simulink model "duplointegrador_2020"  (R2020b)
settings: Solver=ode4  StartTime=0.0  StopTime=30  FixedStep=1e-3  RelTol=1e-3
values from neighbouring files (symbols this model uses):
  N = 4    [duplointegrador_plot_2020.m]
undefined symbols (not defined in the file or in its folder): C, DiscIntNeverNeededParam, Flqr, G, Gamma, h, n, Phi, Q, Q0, Q1, Q2, R, UM, Um, x10, x20, YM, Ym
libraries: simulink x6, eeLuenbergerObserver x1
settings Model: Creator=Trevor  LastModifiedBy=lucas
settings SolverCC: AutoInsertRateTranBlk=on
settings DataIOCC: LimitDataPoints=on  SaveFormat=Array  ReturnWorkspaceOutputs=off
settings OptimizationCC: LifeSpan=inf
settings DebuggingCC: SFUnexpectedBacktrackingDiag=warning  SFNoUnconditionalDefaultTransitionDiag=warning  SFExecutionAtInitializationDiag=none  ArithmeticOperatorsInVariantConditions=warning
settings HardwareCC: ProdBitPerPointer=32  ProdBitPerSizeT=32  ProdBitPerPtrDiffT=32  ProdLargestAtomicFloat=None  ProdIntDivRoundTo=Undefined  ProdEndianess=Unspecified  ProdWordSize=32  ProdHWDeviceType=32-bit Generic
settings ModelReferenceCC: PropagateSignalLabelsOutOfModel=off
settings SFSimCC: SimUseLocalCustomCode=off  CustomCodeUndefinedFunction=UseInterfaceOnly
settings RTWCC: RTWUseLocalCustomCode=off
settings CodeAppCC: StateflowObjectComments=on
settings GRTTargetCC: TargetLangStandard=C89/C90 (ANSI)
settings ConfigComp: CovMetricSettings=dw  CovSaveCumulativeToWorkspaceVar=on  CovSaveSingleToWorkspaceVar=on  CovExternalEMLEnable=off

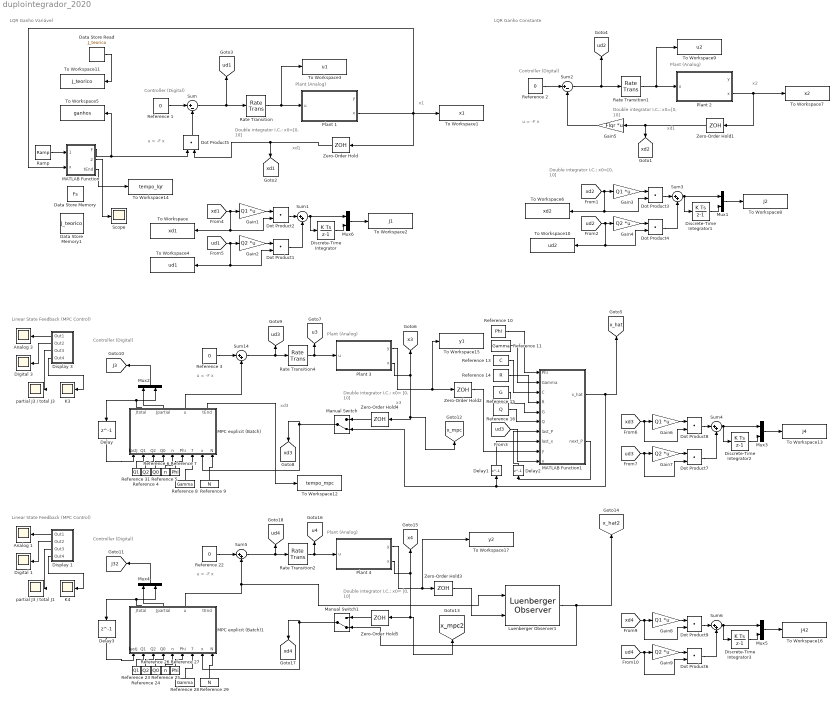
== system duplointegrador_2020 ==
  note: LQR Ganho Constante
  note: LQR Ganho Variável
  note: u = -F x
  note: Double integrator
      | I.C.: x0= [0, 10]
  note: x3
  note: Plant (Analog)
  note: Controller (Digital)
  note: Linear State Feedback (MPC Control)
  note: xd3
  note: u = -F x
  note: Plant (Analog)
  note: x1
  note: Controller (Digital)
  note: Double integrator
      | I.C.: x0=[0, 10]
  note: xd1
  note: Double integrator
      | I.C.: x0=[0, 10]
  note: Controller (Digital)
  note: u = -F x
  note: xd1
  note: x2
  note: Plant (Analog)
  note: Double integrator
      | I.C.: x0=[0, 10]
  note: Double integrator
      | I.C.: x0= [0, 10]
  note: u = -F x
  note: Plant (Analog)
  note: Linear State Feedback (MPC Control)
  note: Controller (Digital)
  Analog 1 : Scope
  Analog 3 : Scope
  Data Store Memory : DataStoreMemory  DataStoreName=Fs  ReadBeforeWriteMsg=warning  WriteAfterWriteMsg=warning  WriteAfterReadMsg=warning  InitialValue=F0  VectorParams1D=off  ShowAdditionalParam=off  OutDataTypeStr=double
  Data Store Memory1 : DataStoreMemory  DataStoreName=J_teorico  ReadBeforeWriteMsg=warning  WriteAfterWriteMsg=warning  WriteAfterReadMsg=warning  VectorParams1D=off  ShowAdditionalParam=off  OutDataTypeStr=double
  Data Store Read : DataStoreRead  DataStoreName=J_teorico
  Delay : Delay  DelayLength=1  SampleTime=h
  Delay1 : Delay  DelayLength=1  InitialCondition=0  SampleTime=h
  Delay2 : Delay  DelayLength=1  InitialCondition=[1 0;0 1]  SampleTime=h
  Delay3 : Delay  DelayLength=1  SampleTime=h
  Digital 1 : Scope
  Digital 3 : Scope
  Discrete-Time Integrator{,1..3} (4 alike) : DiscreteIntegrator  SampleTime=h  ICPrevOutput=DiscIntNeverNeededParam  ICPrevScaledInput=DiscIntNeverNeededParam
  Display 1 : Subsystem
  Display 3 : Subsystem
  Dot Product{1..9} (9 alike) : DotProduct  InputSameDT=on  OutDataTypeStr=Inherit: Inherit via internal rule
  Gain{1,3,6,8} (4 alike) : Gain  Gain=Q1  Multiplication=Matrix(K*u)
  Gain{2,4,7,9} (4 alike) : Gain  Gain=Q2  Multiplication=Matrix(K*u)
  Gain5 : Gain  Gain=Flqr  Multiplication=Matrix(K*u)
  K3 : Scope
  K4 : Scope
  Luenberger Observer1 : eeLuenbergerObserver/Luenberger Observer  StateSpaceType=Discrete-time  Ad=Phi  Bd=Gamma  Cd=C  Dd=D  A=1  B=1  C=1  D=1  ObserverDesign=Desired eigenvalues  Ld=1  DesiredEigenvalues=[0.5, 0.75]  x0=[0, 0]  Tsd=0.1  Ts=-1
      settings: SourceProductBaseCode=PS
  MATLAB Function : MATLAB Function  TreatAsAtomicUnit=on  SystemSampleTime=h
  MATLAB Function1 : MATLAB Function  TreatAsAtomicUnit=on
  MPC explicit (Batch) : MATLAB Function  TreatAsAtomicUnit=on
  MPC explicit (Batch)1 : MATLAB Function  TreatAsAtomicUnit=on
  Manual Switch : ManualSwitch  CurrentSetting=0
  Manual Switch1 : ManualSwitch  CurrentSetting=0
  Mux{1..6} (6 alike) : Mux  Inputs=2
  Plant 1 : Subsystem
      mask Display:
      | text(.5,.6,'dx/dt = Ax + Bu','horizontalAlignment', 'center','verticalAlignment', 'middle','texmode','on')
      | text(.5,.4,'y = Cx + Du','horizontalAlignment', 'center','verticalAlignment', 'middle','texmode','on')
      | port_label('input',1,'u')
      | port_label('output',1,'y')
      | port_label('output',2,'x')
  Plant 2 : Subsystem
      mask Display:
      | text(.5,.6,'dx/dt = Ax + Bu','horizontalAlignment', 'center','verticalAlignment', 'middle','texmode','on')
      | text(.5,.4,'y = Cx + Du','horizontalAlignment', 'center','verticalAlignment', 'middle','texmode','on')
      | port_label('input',1,'u')
      | port_label('output',1,'y')
      | port_label('output',2,'x')
  Plant 3 : Subsystem
      mask Display:
      | text(.5,.6,'dx/dt = Ax + Bu','horizontalAlignment', 'center','verticalAlignment', 'middle','texmode','on')
      | text(.5,.4,'y = Cx + Du','horizontalAlignment', 'center','verticalAlignment', 'middle','texmode','on')
      | port_label('input',1,'u')
      | port_label('output',1,'y')
      | port_label('output',2,'x')
  Plant 4 : Subsystem
      mask Display:
      | text(.5,.6,'dx/dt = Ax + Bu','horizontalAlignment', 'center','verticalAlignment', 'middle','texmode','on')
      | text(.5,.4,'y = Cx + Du','horizontalAlignment', 'center','verticalAlignment', 'middle','texmode','on')
      | port_label('input',1,'u')
      | port_label('output',1,'y')
      | port_label('output',2,'x')
  Ramp : simulink/Sources/Ramp  slope=1  start=0  InitialOutput=0
  Rate Transition : RateTransition  Integrity=off  OutPortSampleTime=h
  Rate Transition1 : RateTransition  Integrity=off  OutPortSampleTime=h
  Rate Transition2 : RateTransition  Integrity=off
  Rate Transition4 : RateTransition  Integrity=off
  Reference {1..3,22} (4 alike) : Constant  Value=0  SampleTime=h
  Reference 10 : Constant  Value=Phi  VectorParams1D=off  SampleTime=h
  Reference 11 : Constant  Value=Gamma  VectorParams1D=off  SampleTime=h
  Reference 13 : Constant  Value=C  VectorParams1D=off  SampleTime=h
  Reference 14 : Constant  Value=R  VectorParams1D=off  SampleTime=h
  Reference 15 : Constant  Value=G  VectorParams1D=off  SampleTime=h
  Reference 16 : Constant  Value=Q  VectorParams1D=off  SampleTime=h
  Reference 23 : Constant  Value=Q1  SampleTime=h
  Reference 24 : Constant  Value=Q2  SampleTime=h
  Reference 25 : Constant  Value=Q0  SampleTime=h
  Reference 26 : Constant  Value=n  SampleTime=h
  Reference 27 : Constant  Value=Phi  SampleTime=h
  Reference 28 : Constant  Value=Gamma  SampleTime=h
  Reference 29 : Constant  Value=N  SampleTime=h
  Reference 31 : Constant  Value=Q1  SampleTime=h
  Reference 4 : Constant  Value=Q2  SampleTime=h
  Reference 5 : Constant  Value=Q0  SampleTime=h
  Reference 6 : Constant  Value=n  SampleTime=h
  Reference 7 : Constant  Value=Phi  SampleTime=h
  Reference 8 : Constant  Value=Gamma  SampleTime=h
  Reference 9 : Constant  Value=N  SampleTime=h
  Scope : Scope
  Sum : Sum  Inputs=|+-
  Sum{1,3..6,14} (6 alike) : Sum  Inputs=|++
  Sum2 : Sum  Inputs=|+-
  To Workspace : ToWorkspace  VariableName=xd1  SaveFormat=Timeseries  SampleTime=h
  To Workspace1 : ToWorkspace  VariableName=x1  SaveFormat=Timeseries  SampleTime=-1
  To Workspace10 : ToWorkspace  VariableName=ud2  SaveFormat=Timeseries  SampleTime=h
  To Workspace11 : ToWorkspace  VariableName=J_teorico  SaveFormat=Timeseries  SampleTime=-1
  To Workspace12 : ToWorkspace  VariableName=tempo_mpc  SaveFormat=Timeseries  SampleTime=h
  To Workspace13 : ToWorkspace  VariableName=J4  SaveFormat=Timeseries  SampleTime=h
  To Workspace14 : ToWorkspace  VariableName=tempo_lqr  SaveFormat=Timeseries  SampleTime=h
  To Workspace15 : ToWorkspace  VariableName=y1  SaveFormat=Timeseries  SampleTime=-1
  To Workspace16 : ToWorkspace  VariableName=J42  SaveFormat=Timeseries  SampleTime=h
  To Workspace17 : ToWorkspace  VariableName=y2  SaveFormat=Timeseries  SampleTime=-1
  To Workspace2 : ToWorkspace  VariableName=J1  SaveFormat=Timeseries  SampleTime=h
  To Workspace3 : ToWorkspace  VariableName=u1  SaveFormat=Timeseries  SampleTime=-1
  To Workspace4 : ToWorkspace  VariableName=ud1  SaveFormat=Timeseries  SampleTime=h
  To Workspace5 : ToWorkspace  VariableName=ganhos  SaveFormat=Timeseries  SampleTime=-1
  To Workspace6 : ToWorkspace  VariableName=xd2  SaveFormat=Timeseries  SampleTime=h
  To Workspace7 : ToWorkspace  VariableName=x2  SaveFormat=Timeseries  SampleTime=-1
  To Workspace8 : ToWorkspace  VariableName=J2  SaveFormat=Timeseries  SampleTime=h
  To Workspace9 : ToWorkspace  VariableName=u2  SaveFormat=Timeseries  SampleTime=-1
  Zero-Order Hold{,1..5} (6 alike) : ZeroOrderHold  SampleTime=h
  partial J3 / total J1 : Scope
  partial J3 / total J3 : Scope
  tag scope: J32=global, J3=global, u3=global, u4=global, ud1=global, ud2=global, ud3=global, ud4=global, x3=global, x4=global, x_hat2=global, x_hat=global, x_mpc2=global, x_mpc=global, xd1=global, xd2=global, xd3=global, xd4=global
  wires:
  Display 3/2(Out2) -> Digital 3/1
  MPC explicit (Batch)/2(Jpartial) -> Mux2/1
  Display 3/4(Out4) -> K3/1
  Reference 5/1 -> MPC explicit (Batch)/4(Q0)
  Display 3/3(Out3) -> partial J3 / total J3/1
  MPC explicit (Batch)/1(Jtotal) -> Delay/1, Mux2/2
  Reference 8/1 -> MPC explicit (Batch)/7(Gamma)
  Plant 3/2(x) -> [x3], [x_mpc], Zero-Order Hold4/1
  Mux2/1 -> [J3]
  Zero-Order Hold4/1 -> Manual Switch/1
  Rate Transition4/1 -> Plant 3/1(u), [u3]
  Reference 4/1 -> MPC explicit (Batch)/3(Q2)
  Delay/1 -> MPC explicit (Batch)/1(lastJ)
  Reference 7/1 -> MPC explicit (Batch)/6(Phi)
  Display 3/1(Out1) -> Analog 3/1
  Reference 6/1 -> MPC explicit (Batch)/5(n)
  Reference 31/1 -> MPC explicit (Batch)/2(Q1)
  Sum14/1 -> [ud3], Rate Transition4/1
  Reference 3/1 -> Sum14/1
  Dot Product1/1 -> Sum1/2
  Data Store Read/1 -> To Workspace11/1
  MATLAB Function/2(indice) -> Scope/1
  Ramp/1 -> MATLAB Function/1(tempo)
  Rate Transition/1 -> Plant 1/1(u), To Workspace3/1
  Reference 1/1 -> Sum/1
  Plant 1/2(x) -> Zero-Order Hold/1, To Workspace1/1, MATLAB Function/2(x)
  Sum/1 -> Rate Transition/1, [ud1]
  Mux6/1 -> To Workspace2/1
  [ud1] -> Gain2/1, Dot Product1/2, To Workspace4/1
  Dot Product5/1 -> Sum/2
  Discrete-Time Integrator/1 -> Mux6/2
  Gain1/1 -> Dot Product2/1
  Sum1/1 -> Discrete-Time Integrator/1, Mux6/1
  Dot Product2/1 -> Sum1/1
  [xd1] -> Dot Product2/2, To Workspace/1, Gain1/1
  Gain2/1 -> Dot Product1/1
  MATLAB Function/1(F) -> To Workspace5/1, Dot Product5/1
  Sum3/1 -> Discrete-Time Integrator1/1, Mux1/1
  Sum2/1 -> Rate Transition1/1, [ud2]
  Zero-Order Hold1/1 -> [xd2], Gain5/1
  Gain5/1 -> Sum2/2
  Dot Product4/1 -> Sum3/2
  Reference 2/1 -> Sum2/1
  Mux1/1 -> To Workspace8/1
  Gain4/1 -> Dot Product4/1
  Dot Product3/1 -> Sum3/1
  [ud2] -> Gain4/1, To Workspace10/1, Dot Product4/2
  Gain3/1 -> Dot Product3/1
  [xd2] -> Dot Product3/2, To Workspace6/1, Gain3/1
  Rate Transition1/1 -> Plant 2/1(u), To Workspace9/1
  Discrete-Time Integrator1/1 -> Mux1/2
  Plant 2/2(x) -> To Workspace7/1, Zero-Order Hold1/1
  Reference 9/1 -> MPC explicit (Batch)/9(N)
  Delay1/1 -> MATLAB Function1/8(last_x)
  MATLAB Function1/1(x_hat) -> [x_hat], Delay1/1, Manual Switch/2
  Plant 3/1(y) -> To Workspace15/1, Zero-Order Hold2/1
  Reference 10/1 -> MATLAB Function1/1(Phi)
  Reference 11/1 -> MATLAB Function1/2(Gamma)
  Reference 13/1 -> MATLAB Function1/3(C)
  Reference 14/1 -> MATLAB Function1/4(R)
  Reference 15/1 -> MATLAB Function1/5(G)
  Reference 16/1 -> MATLAB Function1/6(Q)
  Zero-Order Hold2/1 -> MATLAB Function1/9(y)
  [ud3] -> MATLAB Function1/10(u)
  MATLAB Function1/2(next_P) -> Delay2/1
  Delay2/1 -> MATLAB Function1/7(last_P)
  MPC explicit (Batch)/3(u) -> Sum14/2
  Gain7/1 -> Dot Product7/1
  Gain6/1 -> Dot Product8/1
  Sum4/1 -> Discrete-Time Integrator2/1, Mux3/1
  Dot Product8/1 -> Sum4/1
  Discrete-Time Integrator2/1 -> Mux3/2
  [xd3] -> Dot Product8/2, Gain6/1
  [ud3] -> Gain7/1, Dot Product7/2
  Dot Product7/1 -> Sum4/2
  Mux3/1 -> To Workspace13/1
  MPC explicit (Batch)/4(tEnd) -> To Workspace12/1
  MATLAB Function/3(tEnd) -> To Workspace14/1
  Zero-Order Hold/1 -> [xd1], Dot Product5/2
  Manual Switch/1 -> [xd3], MPC explicit (Batch)/8(x)
  Reference 22/1 -> Sum5/1
  Gain8/1 -> Dot Product9/1
  [xd4] -> Dot Product9/2, Gain8/1
  Reference 26/1 -> MPC explicit (Batch)1/5(n)
  [ud4] -> Gain9/1, Dot Product6/2
  Mux5/1 -> To Workspace16/1
  MPC explicit (Batch)1/2(Jpartial) -> Mux4/1
  Sum6/1 -> Discrete-Time Integrator3/1, Mux5/1
  Dot Product6/1 -> Sum6/2
  MPC explicit (Batch)1/3(u) -> Luenberger Observer1/1, Sum5/2
  Plant 4/2(x) -> [x4], [x_mpc2], Zero-Order Hold5/1
  Discrete-Time Integrator3/1 -> Mux5/2
  Zero-Order Hold5/1 -> Manual Switch1/1
  Manual Switch1/1 -> [xd4], MPC explicit (Batch)1/8(x)
  Dot Product9/1 -> Sum6/1
  Gain9/1 -> Dot Product6/1
  Sum5/1 -> [ud4], Rate Transition2/1
  Display 1/1(Out1) -> Analog 1/1
  Reference 23/1 -> MPC explicit (Batch)1/2(Q1)
  Reference 24/1 -> MPC explicit (Batch)1/3(Q2)
  Delay3/1 -> MPC explicit (Batch)1/1(lastJ)
  Reference 27/1 -> MPC explicit (Batch)1/6(Phi)
  Rate Transition2/1 -> Plant 4/1(u), [u4]
  Reference 29/1 -> MPC explicit (Batch)1/9(N)
  Mux4/1 -> [J32]
  Plant 4/1(y) -> To Workspace17/1, Zero-Order Hold3/1
  Display 1/4(Out4) -> K4/1
  Reference 25/1 -> MPC explicit (Batch)1/4(Q0)
  Reference 28/1 -> MPC explicit (Batch)1/7(Gamma)
  MPC explicit (Batch)1/1(Jtotal) -> Delay3/1, Mux4/2
  Display 1/3(Out3) -> partial J3 / total J1/1
  Display 1/2(Out2) -> Digital 1/1
  Luenberger Observer1/1 -> Manual Switch1/2, [x_hat2]
  Zero-Order Hold3/1 -> Luenberger Observer1/2

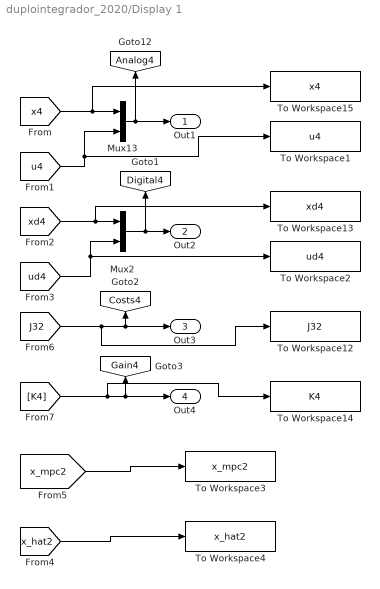
== system duplointegrador_2020/Display 1 ==
  Mux13 : Mux  Inputs=2
  Mux2 : Mux  Inputs=2
  To Workspace1 : ToWorkspace  VariableName=u4  SaveFormat=Timeseries  SampleTime=h
  To Workspace12 : ToWorkspace  VariableName=J32  SaveFormat=Timeseries  SampleTime=h
  To Workspace13 : ToWorkspace  VariableName=xd4  SaveFormat=Timeseries  SampleTime=h
  To Workspace14 : ToWorkspace  VariableName=K4  SaveFormat=Timeseries  SampleTime=h
  To Workspace15 : ToWorkspace  VariableName=x4  SaveFormat=Timeseries  SampleTime=-1
  To Workspace2 : ToWorkspace  VariableName=ud4  SaveFormat=Timeseries  SampleTime=h
  To Workspace3 : ToWorkspace  VariableName=x_mpc2  SaveFormat=Timeseries  SampleTime=-1
  To Workspace4 : ToWorkspace  VariableName=x_hat2  SaveFormat=Timeseries  SampleTime=h
  Out1 : Outport
  Out2 : Outport  Port=2
  Out3 : Outport  Port=3
  Out4 : Outport  Port=4
  tag scope: Analog4=global, Costs4=global, Digital4=global, Gain4=global
  wires:
  Mux13/1 -> Out1/1, [Analog4]
  Mux2/1 -> [Digital4], Out2/1
  [xd4] -> To Workspace13/1, Mux2/1
  [ud4] -> To Workspace2/1, Mux2/2
  [J32] -> To Workspace12/1, [Costs4], Out3/1
  [u4] -> To Workspace1/1, Mux13/2
  [x4] -> To Workspace15/1, Mux13/1
  [K4] -> To Workspace14/1, [Gain4], Out4/1
  [x_mpc2] -> To Workspace3/1
  [x_hat2] -> To Workspace4/1

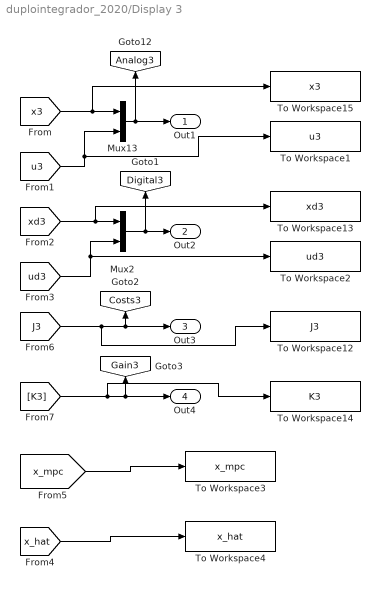
== system duplointegrador_2020/Display 3 ==
  Mux13 : Mux  Inputs=2
  Mux2 : Mux  Inputs=2
  To Workspace1 : ToWorkspace  VariableName=u3  SaveFormat=Timeseries  SampleTime=h
  To Workspace12 : ToWorkspace  VariableName=J3  SaveFormat=Timeseries  SampleTime=h
  To Workspace13 : ToWorkspace  VariableName=xd3  SaveFormat=Timeseries  SampleTime=h
  To Workspace14 : ToWorkspace  VariableName=K3  SaveFormat=Timeseries  SampleTime=h
  To Workspace15 : ToWorkspace  VariableName=x3  SaveFormat=Timeseries  SampleTime=-1
  To Workspace2 : ToWorkspace  VariableName=ud3  SaveFormat=Timeseries  SampleTime=h
  To Workspace3 : ToWorkspace  VariableName=x_mpc  SaveFormat=Timeseries  SampleTime=-1
  To Workspace4 : ToWorkspace  VariableName=x_hat  SaveFormat=Timeseries  SampleTime=h
  Out1 : Outport
  Out2 : Outport  Port=2
  Out3 : Outport  Port=3
  Out4 : Outport  Port=4
  tag scope: Analog3=global, Costs3=global, Digital3=global, Gain3=global
  wires:
  Mux13/1 -> Out1/1, [Analog3]
  Mux2/1 -> [Digital3], Out2/1
  [xd3] -> To Workspace13/1, Mux2/1
  [ud3] -> To Workspace2/1, Mux2/2
  [J3] -> To Workspace12/1, [Costs3], Out3/1
  [u3] -> To Workspace1/1, Mux13/2
  [x3] -> To Workspace15/1, Mux13/1
  [K3] -> To Workspace14/1, [Gain3], Out4/1
  [x_mpc] -> To Workspace3/1
  [x_hat] -> To Workspace4/1

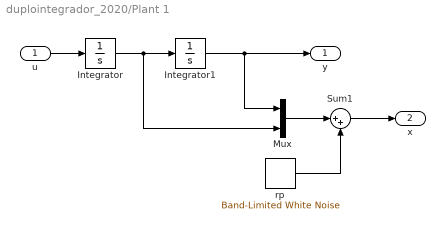
== system duplointegrador_2020/Plant 1 ==
  u : Inport
  Integrator : Integrator  InitialCondition=x10
  Integrator1 : Integrator  InitialCondition=x20
  Mux : Mux  Inputs=2
  Sum1 : Sum  Inputs=|++
  rp : simulink/Sources/Band-Limited White Noise  Cov=rp  Ts=0.001  seed=[23341]
  y : Outport
  x : Outport  Port=2
  wires:
  Integrator/1 -> Mux/2, Integrator1/1
  u/1 -> Integrator/1
  Integrator1/1 -> Mux/1, y/1
  Mux/1 -> Sum1/1
  Sum1/1 -> x/1
  rp/1 -> Sum1/2

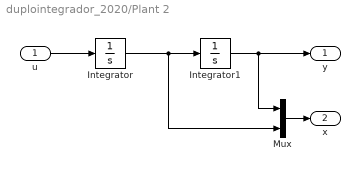
== system duplointegrador_2020/Plant 2 ==
  u : Inport
  Integrator : Integrator  InitialCondition=x10
  Integrator1 : Integrator  InitialCondition=x20
  Mux : Mux  Inputs=2
  y : Outport
  x : Outport  Port=2
  wires:
  Integrator/1 -> Mux/2, Integrator1/1
  Integrator1/1 -> Mux/1, y/1
  u/1 -> Integrator/1
  Mux/1 -> x/1

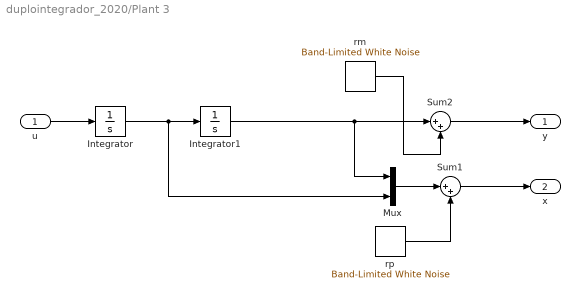
== system duplointegrador_2020/Plant 3 ==
  u : Inport
  Integrator : Integrator  InitialCondition=x10
  Integrator1 : Integrator  InitialCondition=x20
  Mux : Mux  Inputs=2
  Sum1 : Sum  Inputs=|++
  Sum2 : Sum  Inputs=|++
  rm : simulink/Sources/Band-Limited White Noise  Cov=rm  Ts=0.001  seed=[23341]
  rp : simulink/Sources/Band-Limited White Noise  Cov=rp  Ts=0.001  seed=[23341]
  y : Outport
  x : Outport  Port=2
  wires:
  Integrator/1 -> Mux/2, Integrator1/1
  u/1 -> Integrator/1
  Integrator1/1 -> Sum2/1, Mux/1
  Mux/1 -> Sum1/1
  Sum1/1 -> x/1
  rp/1 -> Sum1/2
  Sum2/1 -> y/1
  rm/1 -> Sum2/2

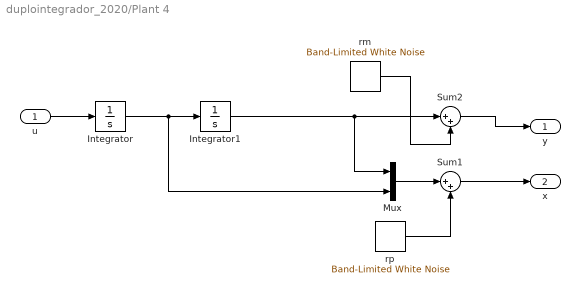
== system duplointegrador_2020/Plant 4 ==
  u : Inport
  Integrator : Integrator  InitialCondition=x10
  Integrator1 : Integrator  InitialCondition=x20
  Mux : Mux  Inputs=2
  Sum1 : Sum  Inputs=|++
  Sum2 : Sum  Inputs=|++
  rm : simulink/Sources/Band-Limited White Noise  Cov=rm  Ts=0.001  seed=[23341]
  rp : simulink/Sources/Band-Limited White Noise  Cov=rp  Ts=0.001  seed=[23341]
  y : Outport
  x : Outport  Port=2
  wires:
  Integrator/1 -> Mux/2, Integrator1/1
  u/1 -> Integrator/1
  Integrator1/1 -> Sum2/1, Mux/1
  Mux/1 -> Sum1/1
  Sum1/1 -> x/1
  rp/1 -> Sum1/2
  rm/1 -> Sum2/2
  Sum2/1 -> y/1

== matlab function duplointegrador_2020/MATLAB Function ==
  settings: updateMethod=DISCRETE
  data: F output; tempo input; n parameter; Q0 parameter; Q2 parameter; Q1 parameter; N parameter; Gamma parameter; Phi parameter; Fs data_store_memory; h parameter; indice output; J_teorico data_store_memory; x input; tEnd output
function [F, indice, tEnd] = LQR(tempo, n, Q0, Q2, Q1, N, Gamma, Phi, h, x)
global Fs J_teorico

tStart = tic;

indice = 1 + mod(floor(tempo/h),N);
if (indice == 1)
    S = zeros(n,n,1,N+1);
    S(:,:,1,N) = Q0;
    for j=(N):-1:1
        S(:,:,1,j) = Phi' * S(:,:,1,j+1) * Phi + Q1 - (Phi' * S(:,:,1,j+1) * Gamma) * inv(Gamma' * S(:,:,1,j+1) * Gamma + Q2) * (Gamma' * S(:,:,1,j+1) * Phi);
        Fs(:,:,1,j) = inv(Q2 + Gamma' * S(:,:,1,j+1) * Gamma) * (Gamma' * S(:,:,1,j+1) * Phi);
    end
    J_teorico = x'*S(:,:,1,1)*x;
end
    
F = Fs(:,:,indice);

tEnd = toc(tStart);

== matlab function duplointegrador_2020/MPC explicit (Batch) ==
  data: Jtotal output; lastJ input; Q1 input; Q2 input; Q0 input; n input; Phi input; Gamma input; x input; Jpartial output; u output; N input; C parameter; UM parameter; Um parameter; YM parameter; Ym parameter; tEnd output
function [Jtotal,Jpartial,u,tEnd] = fcn(lastJ,Q1,Q2,Q0,n,Phi,Gamma,x,N,C,UM, Um, YM, Ym)
%#codegen

tStart = tic;

coder.extrinsic('quadprog');

U = zeros(N,1);
Gain = zeros(2,1);
Jpartial = 0;
Jtotal=0;
fval = 0;
z = zeros(N,1);

M0 = [Phi];
coder.varsize("Mu");
Mu = [Gamma, zeros(size(Gamma,1), N-1)];
Mu_aux = Mu;
Qtil =  kron(eye((N-1)*(n-1)), Q1);
Rbar = kron(eye(N*size(Gamma,2)), Q2);
Qbar = blkdiag(Qtil, Q0);
for i = 1:N-1
    M0 = [M0; Phi^(i+1)];
end
for i = 1:N-1
    Mu_aux = [Mu_aux(1)*Gamma, Mu_aux(:,1:length(Mu_aux)-1)];
    Mu = [Mu; Mu_aux];
end
Qxo = Q1 + M0'*Qbar*M0;
Qu = 2*Mu'*Qbar*Mu + Rbar;
Qxu = 2*M0'*Qbar*Mu;


% %Restrição na entrada
% G_entrada = [eye(N); -eye(N)];
% W_entrada = [UM*ones(N,1);  -Um*ones(N,1)];
% S_entrada = zeros(2*N,n);
% 
% %Restrição na saída(superior)
% G_ss_aux = [Gamma, zeros(n, N-1)]
% G_ss = [C*G_ss_aux]
% for i = 1:N-1
%     G_ss_aux = [Phi*G_ss_aux(1), G_ss_aux(:,1:length(G_ss_aux)-N)]
%     G_ss = [G_ss; C*G_ss_aux]
% end
% W_ss = [YM*ones(N,1)];
% S_si = [C*Phi];
% for i = 1:N-1
%     S_si = [S_si; C*Phi^(i+1)];
% end
% S_ss = -S_si;
% s = [S_entrada; S_ss];
% 
% 
% 
% 
% %Restrição na saída(inferior)
% G_si = -G_ss;
% W_si = [-Ym*ones(N,1)];
% 
% 
% %Parâmetros da função a restrição
% G_teste = [G_si;G_entrada];
% W_teste = [W_si;W_entrada];
% S_teste = [S_si;S_entrada];


[U , fval] = quadprog(2*Qu, 2*Qxu'*x);%, G_teste, W_teste + S_teste*x);
u = U(1,:);
Jpartial =  fval + x'*Qxo*x;
Jtotal = Jpartial+lastJ;

tEnd = toc(tStart);

% G1 = OutroH\OutroF;
% Gain = (evec*G1)';
% u = Gain'*x;
% z = -G1*x;
% Jpartial = 1/2*z'*OutroH*z+x'*OutroF'*z+x'*(Q1+M0'*Qbar*M0)*x;
% Jtotal = Jpartial+lastJ;

== matlab function duplointegrador_2020/MATLAB Function1 ==
  data: Phi input size=[2 2]; Gamma input size=[2 1]; C input size=[1 2]; R input size=1; G input size=[2 1]; Q input size=1; last_P input size=[2 2]; x_hat output size=[2 1]; last_x input size=[2 1]; y input size=1; u input size=1; next_P output size=[2 2]
    function [x_hat, next_P] = fcn(Phi, Gamma, C, R, G, Q, last_P, last_x, y, u)

P = inv(last_P) + C'*inv(R)*C;
P = inv(P);
next_P = Phi*P*Phi' + G*Q*G';
L = P*C'*inv(R);
x = last_x + L*(y - C*last_x);
x_hat = Phi*x + Gamma*u;

== matlab function duplointegrador_2020/MPC explicit (Batch)1 ==
  data: Jtotal output; lastJ input; Q1 input; Q2 input; Q0 input; n input; Phi input; Gamma input; x input; Jpartial output; u output; N input; C parameter; UM parameter; Um parameter; YM parameter; Ym parameter; tEnd output
function [Jtotal,Jpartial,u,tEnd] = fcn(lastJ,Q1,Q2,Q0,n,Phi,Gamma,x,N,C,UM, Um, YM, Ym)
%#codegen

tStart = tic;

coder.extrinsic('quadprog');

U = zeros(N,1);
Gain = zeros(2,1);
Jpartial = 0;
Jtotal=0;
fval = 0;
z = zeros(N,1);

M0 = [Phi];
coder.varsize("Mu");
Mu = [Gamma, zeros(size(Gamma,1), N-1)];
Mu_aux = Mu;
Qtil =  kron(eye((N-1)*(n-1)), Q1);
Rbar = kron(eye(N*size(Gamma,2)), Q2);
Qbar = blkdiag(Qtil, Q0);
for i = 1:N-1
    M0 = [M0; Phi^(i+1)];
end
for i = 1:N-1
    Mu_aux = [Mu_aux(1)*Gamma, Mu_aux(:,1:length(Mu_aux)-1)];
    Mu = [Mu; Mu_aux];
end
Qxo = Q1 + M0'*Qbar*M0;
Qu = 2*Mu'*Qbar*Mu + Rbar;
Qxu = 2*M0'*Qbar*Mu;


% %Restrição na entrada
% G_entrada = [eye(N); -eye(N)];
% W_entrada = [UM*ones(N,1);  -Um*ones(N,1)];
% S_entrada = zeros(2*N,n);
% 
% %Restrição na saída(superior)
% G_ss_aux = [Gamma, zeros(n, N-1)]
% G_ss = [C*G_ss_aux]
% for i = 1:N-1
%     G_ss_aux = [Phi*G_ss_aux(1), G_ss_aux(:,1:length(G_ss_aux)-N)]
%     G_ss = [G_ss; C*G_ss_aux]
% end
% W_ss = [YM*ones(N,1)];
% S_si = [C*Phi];
% for i = 1:N-1
%     S_si = [S_si; C*Phi^(i+1)];
% end
% S_ss = -S_si;
% s = [S_entrada; S_ss];
% 
% 
% 
% 
% %Restrição na saída(inferior)
% G_si = -G_ss;
% W_si = [-Ym*ones(N,1)];
% 
% 
% %Parâmetros da função a restrição
% G_teste = [G_si;G_entrada];
% W_teste = [W_si;W_entrada];
% S_teste = [S_si;S_entrada];


[U , fval] = quadprog(2*Qu, 2*Qxu'*x);%, G_teste, W_teste + S_teste*x);
u = U(1,:);
Jpartial =  fval + x'*Qxo*x;
Jtotal = Jpartial+lastJ;

tEnd = toc(tStart);

% G1 = OutroH\OutroF;
% Gain = (evec*G1)';
% u = Gain'*x;
% z = -G1*x;
% Jpartial = 1/2*z'*OutroH*z+x'*OutroF'*z+x'*(Q1+M0'*Qbar*M0)*x;
% Jtotal = Jpartial+lastJ;
